simulink model "SmartAccess_20221021"  (R2022b)
settings: Solver=FixedStepDiscrete  StartTime=0.0  StopTime=10.0  RelTol=1e-3
undefined symbols (not defined in the file): D1, FrontDriver, Lock, P, UnlockDoor, UnlockDoor_FrontDriver
settings Model: Creator=lcx19  LastModifiedBy=lcx19

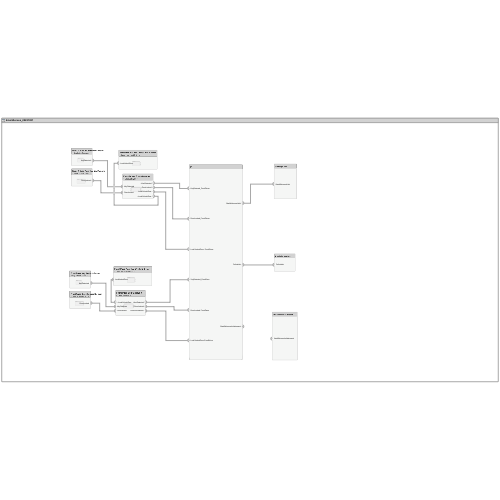
[thumbnail: Simulink's stored preview of the top-level diagram]
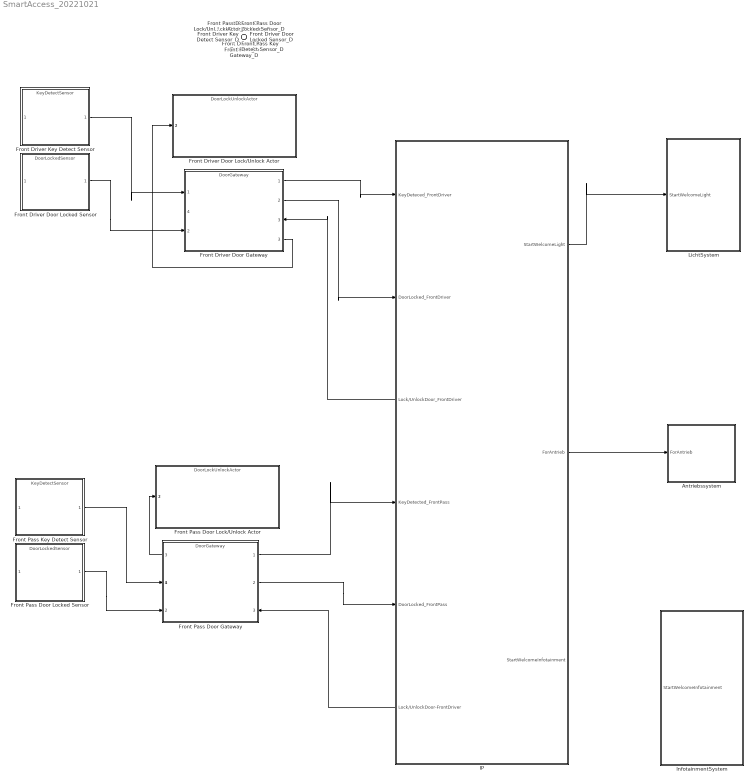
== system SmartAccess_20221021 ==
  Front Driver Door Gateway_D : Inport  OutputFunctionCall=on
  Front Driver Door Lock/Unlock Actor_D : Inport  Port=2  OutputFunctionCall=on
  Front Driver Door Locked Sensor_D : Inport  Port=3  OutputFunctionCall=on
  Front Driver Key Detect Sensor_D : Inport  Port=4  OutputFunctionCall=on
  Front Pass Door Gateway_D : Inport  Port=5  OutputFunctionCall=on
  Front Pass Door Lock/Unlock Actor_D : Inport  Port=6  OutputFunctionCall=on
  Front Pass Door Locked Sensor_D : Inport  Port=7  OutputFunctionCall=on
  Front Pass Key Detect Sensor_D : Inport  Port=8  OutputFunctionCall=on
  Antriebssystem : Subsystem
      settings: PortSchema="{\"entries\":[{\"content\":{\"headerSize\":26,\"margin\":15,\"minimumSpacing\":25,\"sides\":[{\"content\":{\"connectorIds\":[\"In1\"]},\"type\":\"ConnectorPlacement.EquallySpacedRectSide\",\"uuid\":\"97645b60-a3e3-4b43-82f6-27e9bfd07db5\"},{\"content\":{\"connectorIds\":[],\"side\":\"RIGHT\"},\"type\":\"ConnectorPlacement.EquallySpacedRectSide\",\"uuid\":\"7a90ddb5-6793-4894-b93e-cb97d1f1b641\"},{\"content\":{\"connectorIds\":[],\"side\":\"TOP\"},\"type\":\"ConnectorPlacement.EquallySpacedRectSide\",\"uuid\":\"25663444-5f75-44e6-9f0d-ea6311fb2d74\"}]},\"type\":\"ConnectorPlacement.EquallySpacedConnector\",\"uuid\":\"8534c70c-befc-4052-8574-d9dfe944971d\"}],\"packageUris\":[\"http://schema.mathworks.com/mf0/Connector/R2020b\"],\"version\":\"1.0\"}"
  Front Driver Door Gateway : ModelReference  ModelNameDialog=DoorGateway  SimulationMode=Normal  ScheduleRates=on  ModelEventPortInfo=P:D1[-2][0][0]  ModelReferenceVersion=1.6
      settings: PortSchema="{\"entries\":[{\"content\":{\"headerSize\":38,\"margin\":15,\"minimumSpacing\":25,\"sides\":[{\"content\":{\"connectorIds\":[\"In1\",\"In2\"]},\"type\":\"ConnectorPlacement.EquallySpacedRectSide\",\"uuid\":\"f1608663-b487-41b9-a45b-260a442d39bd\"},{\"content\":{\"connectorIds\":[\"Out1\",\"Out2\",\"In3\",\"Out3\"],\"side\":\"RIGHT\"},\"type\":\"ConnectorPlacement.EquallySpacedRectSide\",\"uuid\":\"a744b5c7-61d5-441a-8df7-cb22befe1e9b\"},{\"content\":{\"connectorIds\":[],\"side\":\"TOP\"},\"type\":\"ConnectorPlacement.EquallySpacedRectSide\",\"uuid\":\"c03814ad-5ac5-4a9b-8fc5-ed7f409fe0ba\"},{\"content\":{\"connectorIds\":[\"In4\"],\"side\":\"HIDDEN\"},\"type\":\"ConnectorPlacement.EquallySpacedRectSide\",\"uuid\":\"7344214a-46d4-4b1e-926a-2259fd3ae000\"}]},\"type\":\"ConnectorPlacement.EquallySpacedConnector\",\"uuid\":\"81641bd8-708b-4a10-aaf6-7aaf071f1583\"}],\"packageUris\":[\"http://schema.mathworks.com/mf0/Connector/R2020b\"],\"version\":\"1.0\"}"
  Front Driver Door Lock/Unlock Actor : ModelReference  ModelNameDialog=DoorLockUnlockActor.slx  SimulationMode=Normal  ScheduleRates=on  ModelEventPortInfo=P:D1[-2][0][0]  ModelReferenceVersion=1.2
      settings: PortSchema="{\"entries\":[{\"content\":{\"headerSize\":38,\"margin\":15,\"minimumSpacing\":25,\"sides\":[{\"content\":{\"connectorIds\":[\"In1\"]},\"type\":\"ConnectorPlacement.EquallySpacedRectSide\",\"uuid\":\"f1608663-b487-41b9-a45b-260a442d39bd\"},{\"content\":{\"connectorIds\":[],\"side\":\"RIGHT\"},\"type\":\"ConnectorPlacement.EquallySpacedRectSide\",\"uuid\":\"a744b5c7-61d5-441a-8df7-cb22befe1e9b\"},{\"content\":{\"connectorIds\":[],\"side\":\"TOP\"},\"type\":\"ConnectorPlacement.EquallySpacedRectSide\",\"uuid\":\"c03814ad-5ac5-4a9b-8fc5-ed7f409fe0ba\"},{\"content\":{\"connectorIds\":[\"In2\"],\"side\":\"HIDDEN\"},\"type\":\"ConnectorPlacement.EquallySpacedRectSide\",\"uuid\":\"fd4aa324-5508-485a-a916-ad115134b376\"}]},\"type\":\"ConnectorPlacement.EquallySpacedConnector\",\"uuid\":\"81641bd8-708b-4a10-aaf6-7aaf071f1583\"}],\"packageUris\":[\"http://schema.mathworks.com/mf0/Connector/R2020b\"],\"version\":\"1.0\"}"
  Front Driver Door Locked Sensor : ModelReference  ModelNameDialog=DoorLockedSensor  SimulationMode=Normal  ScheduleRates=on  ModelEventPortInfo=P:D1[-2][0][0]  ModelReferenceVersion=1.1
      settings: PortSchema="{\"entries\":[{\"content\":{\"headerSize\":38,\"margin\":15,\"minimumSpacing\":25,\"sides\":[{\"content\":{\"connectorIds\":[]},\"type\":\"ConnectorPlacement.EquallySpacedRectSide\",\"uuid\":\"f1608663-b487-41b9-a45b-260a442d39bd\"},{\"content\":{\"connectorIds\":[\"Out1\"],\"side\":\"RIGHT\"},\"type\":\"ConnectorPlacement.EquallySpacedRectSide\",\"uuid\":\"a744b5c7-61d5-441a-8df7-cb22befe1e9b\"},{\"content\":{\"connectorIds\":[],\"side\":\"TOP\"},\"type\":\"ConnectorPlacement.EquallySpacedRectSide\",\"uuid\":\"c03814ad-5ac5-4a9b-8fc5-ed7f409fe0ba\"},{\"content\":{\"connectorIds\":[\"In1\"],\"side\":\"HIDDEN\"},\"type\":\"ConnectorPlacement.EquallySpacedRectSide\",\"uuid\":\"62f2e1f5-b023-421c-9fbf-53f0e9727dc5\"}]},\"type\":\"ConnectorPlacement.EquallySpacedConnector\",\"uuid\":\"81641bd8-708b-4a10-aaf6-7aaf071f1583\"}],\"packageUris\":[\"http://schema.mathworks.com/mf0/Connector/R2020b\"],\"version\":\"1.0\"}"
  Front Driver Key Detect Sensor : ModelReference  ModelNameDialog=KeyDetectSensor  SimulationMode=Normal  ScheduleRates=on  ModelEventPortInfo=P:D1[-2][0][0]  ModelReferenceVersion=1.1
      settings: PortSchema="{\"entries\":[{\"content\":{\"headerSize\":38,\"margin\":15,\"minimumSpacing\":25,\"sides\":[{\"content\":{\"connectorIds\":[]},\"type\":\"ConnectorPlacement.EquallySpacedRectSide\",\"uuid\":\"f1608663-b487-41b9-a45b-260a442d39bd\"},{\"content\":{\"connectorIds\":[\"Out1\"],\"side\":\"RIGHT\"},\"type\":\"ConnectorPlacement.EquallySpacedRectSide\",\"uuid\":\"a744b5c7-61d5-441a-8df7-cb22befe1e9b\"},{\"content\":{\"connectorIds\":[],\"side\":\"TOP\"},\"type\":\"ConnectorPlacement.EquallySpacedRectSide\",\"uuid\":\"c03814ad-5ac5-4a9b-8fc5-ed7f409fe0ba\"},{\"content\":{\"connectorIds\":[\"In1\"],\"side\":\"HIDDEN\"},\"type\":\"ConnectorPlacement.EquallySpacedRectSide\",\"uuid\":\"b8e44f42-a3e2-43a8-a16d-0715ca6ed244\"}]},\"type\":\"ConnectorPlacement.EquallySpacedConnector\",\"uuid\":\"81641bd8-708b-4a10-aaf6-7aaf071f1583\"}],\"packageUris\":[\"http://schema.mathworks.com/mf0/Connector/R2020b\"],\"version\":\"1.0\"}"
  Front Pass Door Gateway : ModelReference  ModelNameDialog=DoorGateway  SimulationMode=Normal  ScheduleRates=on  ModelEventPortInfo=P:D1[-2][0][0]  ModelReferenceVersion=1.6
      settings: PortSchema="{\"entries\":[{\"content\":{\"headerSize\":38,\"margin\":15,\"minimumSpacing\":25,\"sides\":[{\"content\":{\"connectorIds\":[\"Out3\",\"In1\",\"In2\"]},\"type\":\"ConnectorPlacement.EquallySpacedRectSide\",\"uuid\":\"f1608663-b487-41b9-a45b-260a442d39bd\"},{\"content\":{\"connectorIds\":[\"Out1\",\"Out2\",\"In3\"],\"side\":\"RIGHT\"},\"type\":\"ConnectorPlacement.EquallySpacedRectSide\",\"uuid\":\"a744b5c7-61d5-441a-8df7-cb22befe1e9b\"},{\"content\":{\"connectorIds\":[],\"side\":\"TOP\"},\"type\":\"ConnectorPlacement.EquallySpacedRectSide\",\"uuid\":\"c03814ad-5ac5-4a9b-8fc5-ed7f409fe0ba\"},{\"content\":{\"connectorIds\":[\"In4\"],\"side\":\"HIDDEN\"},\"type\":\"ConnectorPlacement.EquallySpacedRectSide\",\"uuid\":\"2bd42873-1ccb-4f73-9649-67148e1da346\"}]},\"type\":\"ConnectorPlacement.EquallySpacedConnector\",\"uuid\":\"81641bd8-708b-4a10-aaf6-7aaf071f1583\"}],\"packageUris\":[\"http://schema.mathworks.com/mf0/Connector/R2020b\"],\"version\":\"1.0\"}"
  Front Pass Door Lock/Unlock Actor : ModelReference  ModelNameDialog=DoorLockUnlockActor.slx  SimulationMode=Normal  ScheduleRates=on  ModelEventPortInfo=P:D1[-2][0][0]  ModelReferenceVersion=1.2
      settings: PortSchema="{\"entries\":[{\"content\":{\"headerSize\":38,\"margin\":15,\"minimumSpacing\":25,\"sides\":[{\"content\":{\"connectorIds\":[\"In1\"]},\"type\":\"ConnectorPlacement.EquallySpacedRectSide\",\"uuid\":\"f1608663-b487-41b9-a45b-260a442d39bd\"},{\"content\":{\"connectorIds\":[],\"side\":\"RIGHT\"},\"type\":\"ConnectorPlacement.EquallySpacedRectSide\",\"uuid\":\"a744b5c7-61d5-441a-8df7-cb22befe1e9b\"},{\"content\":{\"connectorIds\":[],\"side\":\"TOP\"},\"type\":\"ConnectorPlacement.EquallySpacedRectSide\",\"uuid\":\"c03814ad-5ac5-4a9b-8fc5-ed7f409fe0ba\"},{\"content\":{\"connectorIds\":[\"In2\"],\"side\":\"HIDDEN\"},\"type\":\"ConnectorPlacement.EquallySpacedRectSide\",\"uuid\":\"fd4aa324-5508-485a-a916-ad115134b376\"}]},\"type\":\"ConnectorPlacement.EquallySpacedConnector\",\"uuid\":\"81641bd8-708b-4a10-aaf6-7aaf071f1583\"}],\"packageUris\":[\"http://schema.mathworks.com/mf0/Connector/R2020b\"],\"version\":\"1.0\"}"
  Front Pass Door Locked Sensor : ModelReference  ModelNameDialog=DoorLockedSensor  SimulationMode=Normal  ScheduleRates=on  ModelEventPortInfo=P:D1[-2][0][0]  ModelReferenceVersion=1.1
      settings: PortSchema="{\"entries\":[{\"content\":{\"headerSize\":38,\"margin\":15,\"minimumSpacing\":25,\"sides\":[{\"content\":{\"connectorIds\":[]},\"type\":\"ConnectorPlacement.EquallySpacedRectSide\",\"uuid\":\"f1608663-b487-41b9-a45b-260a442d39bd\"},{\"content\":{\"connectorIds\":[\"Out1\"],\"side\":\"RIGHT\"},\"type\":\"ConnectorPlacement.EquallySpacedRectSide\",\"uuid\":\"a744b5c7-61d5-441a-8df7-cb22befe1e9b\"},{\"content\":{\"connectorIds\":[],\"side\":\"TOP\"},\"type\":\"ConnectorPlacement.EquallySpacedRectSide\",\"uuid\":\"c03814ad-5ac5-4a9b-8fc5-ed7f409fe0ba\"},{\"content\":{\"connectorIds\":[\"In1\"],\"side\":\"HIDDEN\"},\"type\":\"ConnectorPlacement.EquallySpacedRectSide\",\"uuid\":\"6d6bc871-ea03-41b9-90b5-59ec9cc532dc\"}]},\"type\":\"ConnectorPlacement.EquallySpacedConnector\",\"uuid\":\"81641bd8-708b-4a10-aaf6-7aaf071f1583\"}],\"packageUris\":[\"http://schema.mathworks.com/mf0/Connector/R2020b\"],\"version\":\"1.0\"}"
  Front Pass Key Detect Sensor : ModelReference  ModelNameDialog=KeyDetectSensor  SimulationMode=Normal  ScheduleRates=on  ModelEventPortInfo=P:D1[-2][0][0]  ModelReferenceVersion=1.1
      settings: PortSchema="{\"entries\":[{\"content\":{\"headerSize\":38,\"margin\":15,\"minimumSpacing\":25,\"sides\":[{\"content\":{\"connectorIds\":[]},\"type\":\"ConnectorPlacement.EquallySpacedRectSide\",\"uuid\":\"f1608663-b487-41b9-a45b-260a442d39bd\"},{\"content\":{\"connectorIds\":[\"Out1\"],\"side\":\"RIGHT\"},\"type\":\"ConnectorPlacement.EquallySpacedRectSide\",\"uuid\":\"a744b5c7-61d5-441a-8df7-cb22befe1e9b\"},{\"content\":{\"connectorIds\":[],\"side\":\"TOP\"},\"type\":\"ConnectorPlacement.EquallySpacedRectSide\",\"uuid\":\"c03814ad-5ac5-4a9b-8fc5-ed7f409fe0ba\"},{\"content\":{\"connectorIds\":[\"In1\"],\"side\":\"HIDDEN\"},\"type\":\"ConnectorPlacement.EquallySpacedRectSide\",\"uuid\":\"85a5aa8b-cb09-4196-b955-fbfa1b15b1f9\"}]},\"type\":\"ConnectorPlacement.EquallySpacedConnector\",\"uuid\":\"81641bd8-708b-4a10-aaf6-7aaf071f1583\"}],\"packageUris\":[\"http://schema.mathworks.com/mf0/Connector/R2020b\"],\"version\":\"1.0\"}"
  IP : Subsystem
      settings: PortSchema="{\"entries\":[{\"content\":{\"headerSize\":26,\"margin\":15,\"minimumSpacing\":25,\"sides\":[{\"content\":{\"connectorIds\":[\"In1\",\"In2\",\"Out4\",\"In3\",\"In4\",\"Out5\"]},\"type\":\"ConnectorPlacement.EquallySpacedRectSide\",\"uuid\":\"97645b60-a3e3-4b43-82f6-27e9bfd07db5\"},{\"content\":{\"connectorIds\":[\"Out1\",\"Out2\",\"Out3\"],\"side\":\"RIGHT\"},\"type\":\"ConnectorPlacement.EquallySpacedRectSide\",\"uuid\":\"7a90ddb5-6793-4894-b93e-cb97d1f1b641\"},{\"content\":{\"connectorIds\":[],\"side\":\"TOP\"},\"type\":\"ConnectorPlacement.EquallySpacedRectSide\",\"uuid\":\"25663444-5f75-44e6-9f0d-ea6311fb2d74\"}]},\"type\":\"ConnectorPlacement.EquallySpacedConnector\",\"uuid\":\"8534c70c-befc-4052-8574-d9dfe944971d\"}],\"packageUris\":[\"http://schema.mathworks.com/mf0/Connector/R2020b\"],\"version\":\"1.0\"}"
  InfotainmentSystem : Subsystem
      settings: PortSchema="{\"entries\":[{\"content\":{\"headerSize\":26,\"margin\":15,\"minimumSpacing\":25,\"sides\":[{\"content\":{\"connectorIds\":[\"In1\"]},\"type\":\"ConnectorPlacement.EquallySpacedRectSide\",\"uuid\":\"97645b60-a3e3-4b43-82f6-27e9bfd07db5\"},{\"content\":{\"connectorIds\":[],\"side\":\"RIGHT\"},\"type\":\"ConnectorPlacement.EquallySpacedRectSide\",\"uuid\":\"7a90ddb5-6793-4894-b93e-cb97d1f1b641\"},{\"content\":{\"connectorIds\":[],\"side\":\"TOP\"},\"type\":\"ConnectorPlacement.EquallySpacedRectSide\",\"uuid\":\"25663444-5f75-44e6-9f0d-ea6311fb2d74\"}]},\"type\":\"ConnectorPlacement.EquallySpacedConnector\",\"uuid\":\"8534c70c-befc-4052-8574-d9dfe944971d\"}],\"packageUris\":[\"http://schema.mathworks.com/mf0/Connector/R2020b\"],\"version\":\"1.0\"}"
  LichtSystem : Subsystem
      settings: PortSchema="{\"entries\":[{\"content\":{\"headerSize\":26,\"margin\":15,\"minimumSpacing\":25,\"sides\":[{\"content\":{\"connectorIds\":[\"In1\"]},\"type\":\"ConnectorPlacement.EquallySpacedRectSide\",\"uuid\":\"97645b60-a3e3-4b43-82f6-27e9bfd07db5\"},{\"content\":{\"connectorIds\":[],\"side\":\"RIGHT\"},\"type\":\"ConnectorPlacement.EquallySpacedRectSide\",\"uuid\":\"7a90ddb5-6793-4894-b93e-cb97d1f1b641\"},{\"content\":{\"connectorIds\":[],\"side\":\"TOP\"},\"type\":\"ConnectorPlacement.EquallySpacedRectSide\",\"uuid\":\"25663444-5f75-44e6-9f0d-ea6311fb2d74\"}]},\"type\":\"ConnectorPlacement.EquallySpacedConnector\",\"uuid\":\"8534c70c-befc-4052-8574-d9dfe944971d\"}],\"packageUris\":[\"http://schema.mathworks.com/mf0/Connector/R2020b\"],\"version\":\"1.0\"}"
  wires:
  Front Driver Key Detect Sensor/1 -> Front Driver Door Gateway/1
  Front Driver Door Locked Sensor/1 -> Front Driver Door Gateway/2
  IP/4(Lock/UnlockDoor_FrontDriver) -> Front Driver Door Gateway/3
  Front Pass Key Detect Sensor/1 -> Front Pass Door Gateway/1
  Front Pass Door Locked Sensor/1 -> Front Pass Door Gateway/2
  Front Driver Door Gateway/3 -> Front Driver Door Lock/Unlock Actor/1
  Front Driver Door Gateway/1 -> IP/1(KeyDeteced_FrontDriver)
  Front Driver Door Gateway/2 -> IP/2(DoorLocked_FrontDriver)
  Front Pass Door Gateway/1 -> IP/3(KeyDetected_FrontPass)
  Front Pass Door Gateway/2 -> IP/4(DoorLocked_FrontPass)
  IP/5(Lock/UnlockDoor-FrontDriver) -> Front Pass Door Gateway/3
  Front Pass Door Gateway/3 -> Front Pass Door Lock/Unlock Actor/1
  IP/2(ForAntrieb) -> Antriebssystem/1(ForAntrieb)
  IP/1(StartWelcomeLight) -> LichtSystem/1(StartWelcomeLight)

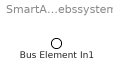
== system SmartAccess_20221021/Antriebssystem ==
  Bus Element In1 : Inport  PortName=ForAntrieb

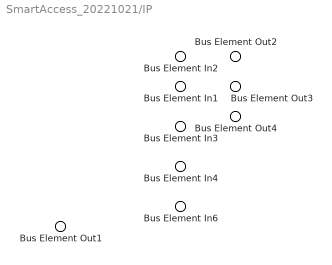
== system SmartAccess_20221021/IP ==
  Bus Element In1 : Inport  PortName=KeyDeteced_FrontDriver
  Bus Element In2 : Inport  Port=2  PortName=DoorLocked_FrontDriver
  Bus Element In3 : Inport  Port=3  PortName=KeyDetected_FrontPass
  Bus Element In4 : Inport  Port=4  PortName=DoorLocked_FrontPass
  Bus Element Out3 : Outport  PortName=StartWelcomeLight
  Bus Element Out2 : Outport  Port=2  PortName=ForAntrieb
  Bus Element Out4 : Outport  Port=3  PortName=StartWelcomeInfotainment
  Bus Element Out1 : Outport  Port=4  PortName=Lock/UnlockDoor_FrontDriver
  Bus Element In6 : Outport  Port=5  PortName=Lock/UnlockDoor-FrontDriver

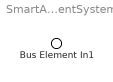
== system SmartAccess_20221021/InfotainmentSystem ==
  Bus Element In1 : Inport  PortName=StartWelcomeInfotainment

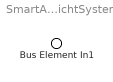
== system SmartAccess_20221021/LichtSystem ==
  Bus Element In1 : Inport  PortName=StartWelcomeLight
